simulink model "vocoder_v1"  (R2020a)
settings: Solver=FixedStepDiscrete  StartTime=0.0  StopTime=inf  RelTol=1e-3
libraries: audiosources x2, dspsnks4 x1, audiofilters x1
settings Model: Creator=unity  LastModifiedBy=unity
settings SolverCC: AutoInsertRateTranBlk=on
settings DataIOCC: LimitDataPoints=on  SaveOutput=off  SignalLogging=off  SaveTime=off
settings OptimizationCC: LifeSpan=inf
settings DebuggingCC: AlgebraicLoopMsg=error  SingleTaskRateTransMsg=error  AllowSymbolicDim=off  SFUnexpectedBacktrackingDiag=warning  SFNoUnconditionalDefaultTransitionDiag=warning  SFExecutionAtInitializationDiag=none  ArithmeticOperatorsInVariantConditions=warning
settings SFSimCC: SimUseLocalCustomCode=off  CustomCodeUndefinedFunction=UseInterfaceOnly
settings RTWCC: RTWUseLocalCustomCode=off
settings CodeAppCC: StateflowObjectComments=on
settings GRTTargetCC: TargetLangStandard=C89/C90 (ANSI)
settings ConfigComp: CovMetricSettings=dw  CovHtmlReporting=on  CovSaveCumulativeToWorkspaceVar=on  CovSaveSingleToWorkspaceVar=on  CovExternalEMLEnable=off  CovSFcnEnable=off

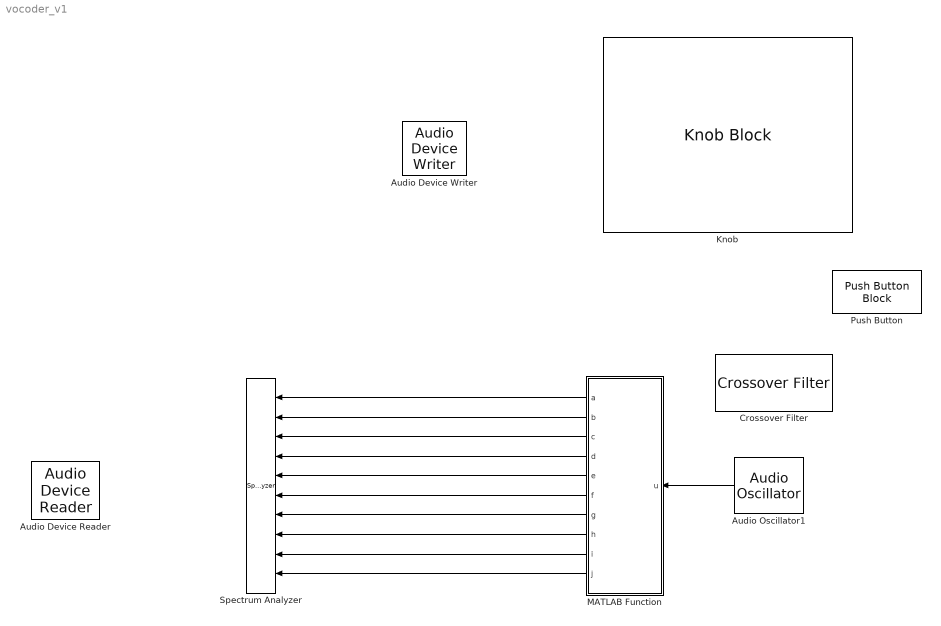
== system vocoder_v1 ==
  Audio Device Reader : audiosources/Audio Device Reader  Driver=DirectSound  Device=Default  SampleRate=44100  NumChannels=1  SamplesPerFrame=1024  BitDepth=16-bit integer  NumBuffers=10  DefaultInputChannelMapping=on  InputChannelMapping=1:2  OutputNumOverrunSamples=off  OutputDataType=double  DriverIdx=1  DeviceWarnFlag=''
      settings: SourceProductBaseCode=AU
  Audio Device Writer : dspsnks4/Audio Device Writer  Driver=DirectSound  Device=Default  InheritSampleRate=on  SampleRate=44100  BitDepth=16-bit integer  BufferSize=4096  NumBuffers=10  DefaultOutputChannelMapping=on  OutputChannelMapping=1:2  OutputNumUnderrunSamples=off  DriverIdx=1  DeviceWarnFlag=''
  Audio Oscillator1 : audiosources/Audio Oscillator  FrequencyPort=off  Frequency=150  AmplitudePort=off  Amplitude=1  DCOffsetPort=off  PhaseOffset=0  DCOffset=0  WidthPort=off  Width=1  DutyCyclePort=off  DutyCycle=0.5  SampsPerFrame=1024  Fs=44100  OutputDataType=double  SimulateUsing=Code generation
      settings: SourceProductBaseCode=AU  SignalType=sawtooth
  Crossover Filter : audiofilters/Crossover Filter  NCrossovers=1  Crossover1Port=off  Crossover1=100  Order1Port=off  Order1=2  Crossover2Port=off  Crossover2=800  Order2Port=off  Order2=2  Crossover3Port=off  Crossover3=1500  Order3Port=off  Order3=2  Crossover4Port=off  Crossover4=3000  Order4Port=off  Order4=2  InheritSampleRate=off  SampleRate=44100  SimulateUsing=Code generation
      settings: SourceProductBaseCode=AU
  Knob : KnobBlock  ScaleMin=20  ScaleMax=20000  ScaleType=Log
  MATLAB Function : MATLAB Function  TreatAsAtomicUnit=on
  Push Button : PushButtonBlock
  Spectrum Analyzer : SpectrumAnalyzer  NumInputPorts=10
  wires:
  Audio Oscillator1/1 -> MATLAB Function/1(u)
  MATLAB Function/1(a) -> Spectrum Analyzer/1
  MATLAB Function/2(b) -> Spectrum Analyzer/2
  MATLAB Function/3(c) -> Spectrum Analyzer/3
  MATLAB Function/4(d) -> Spectrum Analyzer/4
  MATLAB Function/5(e) -> Spectrum Analyzer/5
  MATLAB Function/6(f) -> Spectrum Analyzer/6
  MATLAB Function/7(g) -> Spectrum Analyzer/7
  MATLAB Function/8(h) -> Spectrum Analyzer/8
  MATLAB Function/9(i) -> Spectrum Analyzer/9
  MATLAB Function/10(j) -> Spectrum Analyzer/10

== matlab function vocoder_v1/MATLAB Function ==
  data: u input; a output; b output; c output; d output; e output; f output; g output; h output; i output; j output
function [a,b,c,d,e,f,g,h,i,j] = fcn(u) 
    
    min = 80;
    max = 8000;
    n = 10;
    bands = 1:n;
    freqs = min*(max/min).^((bands-1)/(n-1));
    
    Fs = 44.1e3; 
    filtertype = 'FIR';
    Fpass = freqs/1.1;
    Fstop = freqs*1.1; 
    Rp = 0.1;
    Astop = 80;
    
    persistent filters
    
    if isempty(filters)
        filters = {dsp.LowpassFilter('SampleRate',Fs, ...
             'FilterType',filtertype, ...
             'PassbandFrequency',Fpass(1), ...
             'StopbandFrequency',Fstop(1), ...
             'PassbandRipple',Rp, ...
             'StopbandAttenuation',Astop),dsp.LowpassFilter(),
             dsp.LowpassFilter('SampleRate',Fs, ...
             'FilterType',filtertype, ...
             'PassbandFrequency',Fpass(2), ...
             'StopbandFrequency',Fstop(2), ...
             'PassbandRipple',Rp, ...
             'StopbandAttenuation',Astop),dsp.LowpassFilter(),
             dsp.LowpassFilter('SampleRate',Fs, ...
             'FilterType',filtertype, ...
             'PassbandFrequency',Fpass(3), ...
             'StopbandFrequency',Fstop(3), ...
             'PassbandRipple',Rp, ...
             'StopbandAttenuation',Astop),dsp.LowpassFilter(),
             dsp.LowpassFilter('SampleRate',Fs, ...
             'FilterType',filtertype, ...
             'PassbandFrequency',Fpass(4), ...
             'StopbandFrequency',Fstop(4), ...
             'PassbandRipple',Rp, ...
             'StopbandAttenuation',Astop),dsp.LowpassFilter(),
             dsp.LowpassFilter('SampleRate',Fs, ...
             'FilterType',filtertype, ...
             'PassbandFrequency',Fpass(5), ...
             'StopbandFrequency',Fstop(5), ...
             'PassbandRipple',Rp, ...
             'StopbandAttenuation',Astop),dsp.LowpassFilter(),
             dsp.LowpassFilter('SampleRate',Fs, ...
             'FilterType',filtertype, ...
             'PassbandFrequency',Fpass(6), ...
             'StopbandFrequency',Fstop(6), ...
             'PassbandRipple',Rp, ...
             'StopbandAttenuation',Astop),dsp.LowpassFilter(),
             dsp.LowpassFilter('SampleRate',Fs, ...
             'FilterType',filtertype, ...
             'PassbandFrequency',Fpass(7), ...
             'StopbandFrequency',Fstop(7), ...
             'PassbandRipple',Rp, ...
             'StopbandAttenuation',Astop),dsp.LowpassFilter(),
             dsp.LowpassFilter('SampleRate',Fs, ...
             'FilterType',filtertype, ...
             'PassbandFrequency',Fpass(8), ...
             'StopbandFrequency',Fstop(8), ...
             'PassbandRipple',Rp, ...
             'StopbandAttenuation',Astop),dsp.LowpassFilter(),
             dsp.LowpassFilter('SampleRate',Fs, ...
             'FilterType',filtertype, ...
             'PassbandFrequency',Fpass(9), ...
             'StopbandFrequency',Fstop(9), ...
             'PassbandRipple',Rp, ...
             'StopbandAttenuation',Astop),dsp.LowpassFilter(),
             dsp.LowpassFilter('SampleRate',Fs, ...
             'FilterType',filtertype, ...
             'PassbandFrequency',Fpass(10), ...
             'StopbandFrequency',Fstop(10), ...
             'PassbandRipple',Rp, ...
             'StopbandAttenuation',Astop),dsp.LowpassFilter(),};
    end
    

    a=filters{1}(u);
    b=filters{2}(u);
    c=filters{3}(u);
    d=filters{4}(u);
    e=filters{5}(u);
    f=filters{6}(u);
    g=filters{7}(u);
    h=filters{8}(u);
    i=filters{9}(u);
    j=filters{10}(u);
